simulink model "simu"  (R2021a)
settings: Solver=FixedStepAuto  StartTime=0.0  StopTime=3600  FixedStep=1  RelTol=1e-3
libraries: fuzblock x4
settings Model: Creator=Ana  LastModifiedBy=Ana

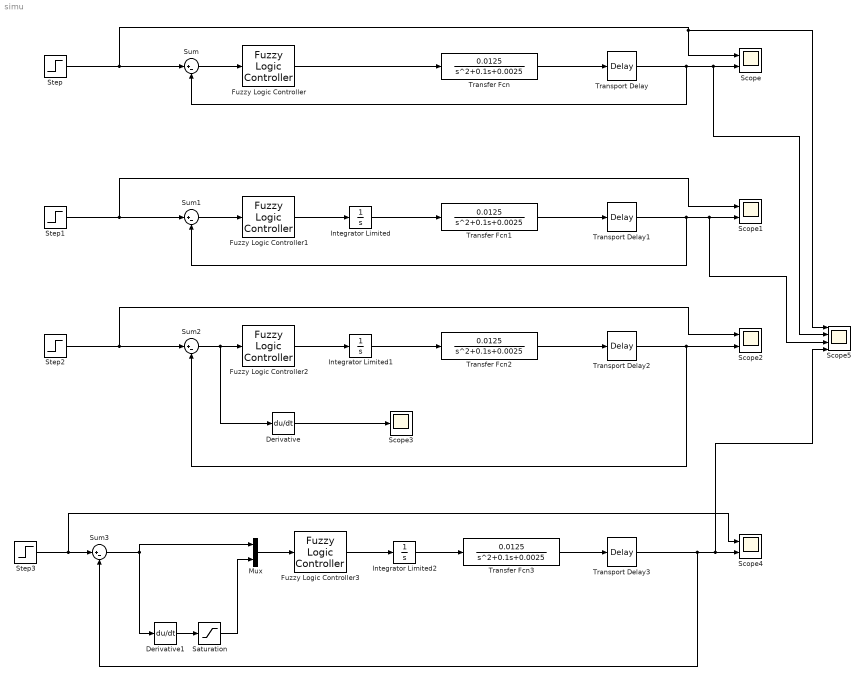
== system simu ==
  Derivative : Derivative
  Derivative1 : Derivative
  Fuzzy Logic Controller : fuzblock/Fuzzy Logic  Controller  FIS='proj2.fis'  OutputSampleNumber=101  DataType=double  FuzzifiedInputs=off  RuleFiringStrengths=off  RuleOutputs=off  AggregatedOutputs=off  SimulateUsing=Interpreted execution  OutOfRangeInputValueMessage=warning  NoRuleFiredMessage=warning  EmptyOutputFuzzySetMessage=warning
  Fuzzy Logic Controller1 : fuzblock/Fuzzy Logic  Controller  FIS='proj2.1.fis'  OutputSampleNumber=101  DataType=double  FuzzifiedInputs=off  RuleFiringStrengths=off  RuleOutputs=off  AggregatedOutputs=off  SimulateUsing=Interpreted execution  OutOfRangeInputValueMessage=warning  NoRuleFiredMessage=warning  EmptyOutputFuzzySetMessage=warning
  Fuzzy Logic Controller2 : fuzblock/Fuzzy Logic  Controller  FIS='proj2.1.fis'  OutputSampleNumber=101  DataType=double  FuzzifiedInputs=off  RuleFiringStrengths=off  RuleOutputs=off  AggregatedOutputs=off  SimulateUsing=Interpreted execution  OutOfRangeInputValueMessage=warning  NoRuleFiredMessage=warning  EmptyOutputFuzzySetMessage=warning
  Fuzzy Logic Controller3 : fuzblock/Fuzzy Logic  Controller  FIS='proj2.2.fis'  OutputSampleNumber=101  DataType=double  FuzzifiedInputs=off  RuleFiringStrengths=off  RuleOutputs=off  AggregatedOutputs=off  SimulateUsing=Interpreted execution  OutOfRangeInputValueMessage=warning  NoRuleFiredMessage=warning  EmptyOutputFuzzySetMessage=warning
  Integrator Limited : Integrator  LimitOutput=on  UpperSaturationLimit=0.5  LowerSaturationLimit=-0.5
  Integrator Limited1 : Integrator  LimitOutput=on  UpperSaturationLimit=0.5  LowerSaturationLimit=-0.5
  Integrator Limited2 : Integrator  LimitOutput=on  UpperSaturationLimit=0.5  LowerSaturationLimit=-0.5
  Mux : Mux  Inputs=2
  Saturation : Saturate  UpperLimit=0.02  LowerLimit=-0.02
  Scope{,1..2,4} (4 alike) : Scope  NumInputPorts=2
  Scope3 : Scope
  Scope5 : Scope  NumInputPorts=4
  Step{,1..3} (4 alike) : Step  Time=1000  Before=-2  After=2  SampleTime=0
  Sum{,1..3} (4 alike) : Sum  Inputs=|+-
  Transfer Fcn{,1..3} (4 alike) : TransferFcn  Numerator=[0.0125]  Denominator=[1 0.1 0.0025]
  Transport Delay{,1..3} (4 alike) : TransportDelay  DelayTime=8
  wires:
  Transfer Fcn/1 -> Transport Delay/1
  Sum/1 -> Fuzzy Logic Controller/1
  Fuzzy Logic Controller/1 -> Transfer Fcn/1
  Step/1 -> Scope/1, Scope5/1, Sum/1
  Transport Delay/1 -> Sum/2, Scope5/2, Scope/2
  Sum1/1 -> Fuzzy Logic Controller1/1
  Transport Delay1/1 -> Sum1/2, Scope5/3, Scope1/2
  Step1/1 -> Scope1/1, Sum1/1
  Transfer Fcn1/1 -> Transport Delay1/1
  Fuzzy Logic Controller1/1 -> Integrator Limited/1
  Integrator Limited/1 -> Transfer Fcn1/1
  Fuzzy Logic Controller2/1 -> Integrator Limited1/1
  Integrator Limited1/1 -> Transfer Fcn2/1
  Transfer Fcn2/1 -> Transport Delay2/1
  Step2/1 -> Scope2/1, Sum2/1
  Transport Delay2/1 -> Sum2/2, Scope2/2
  Sum2/1 -> Derivative/1, Fuzzy Logic Controller2/1
  Derivative/1 -> Scope3/1
  Sum3/1 -> Mux/1, Derivative1/1
  Transport Delay3/1 -> Scope4/2, Scope5/4, Sum3/2
  Integrator Limited2/1 -> Transfer Fcn3/1
  Transfer Fcn3/1 -> Transport Delay3/1
  Step3/1 -> Scope4/1, Sum3/1
  Fuzzy Logic Controller3/1 -> Integrator Limited2/1
  Mux/1 -> Fuzzy Logic Controller3/1
  Derivative1/1 -> Saturation/1
  Saturation/1 -> Mux/2
